simulink model "Series_Parallel_HEV_PowerFlow_Simulink"  (R2024b)
settings: Solver=VariableStepAuto  StartTime=0.0  StopTime=15  RelTol=1e-3
libraries: simulink x3
settings Model: Creator=JAMES  LastModifiedBy=JAMES

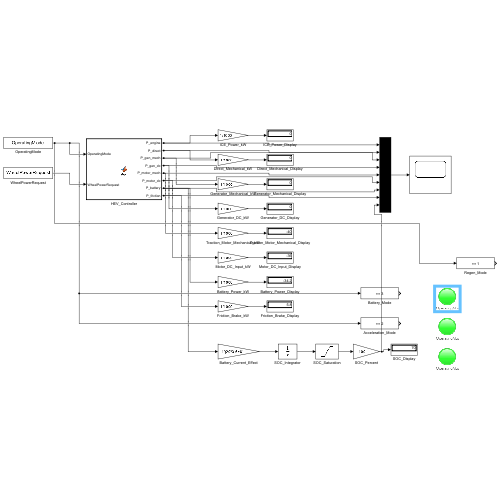
[thumbnail: Simulink's stored preview of the top-level diagram]
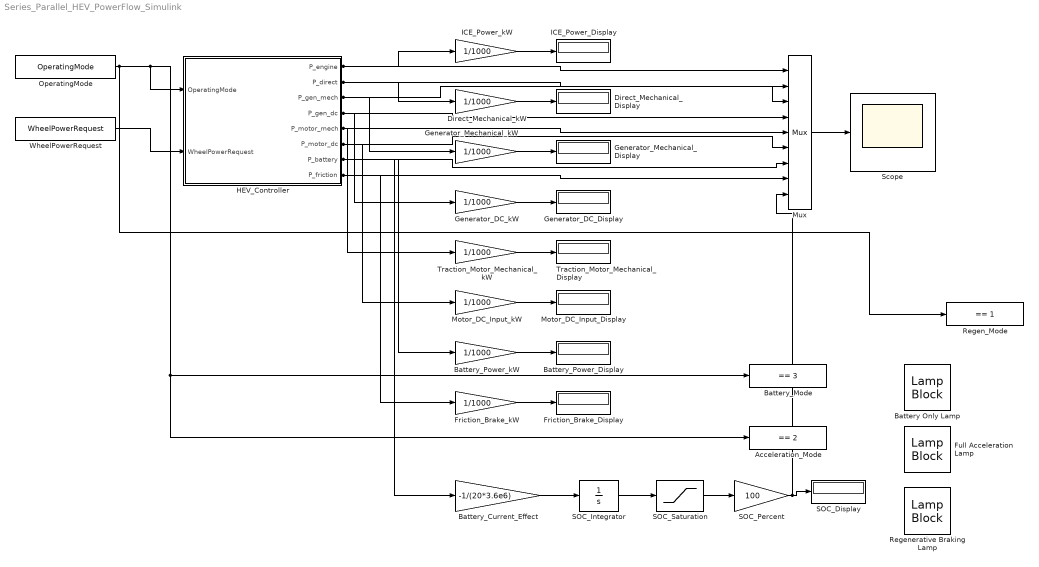
== system Series_Parallel_HEV_PowerFlow_Simulink ==
  Acceleration_Mode : simulink/Logic and Bit Operations/Compare To Constant  relop===  const=2  OutDataTypeStr=boolean
  Battery Only Lamp : LampBlock  LabelPosition=Bottom
  Battery_Current_Effect : Gain  Gain=-1/(20*3.6e6)
  Battery_Mode : simulink/Logic and Bit Operations/Compare To Constant  relop===  const=3  OutDataTypeStr=boolean
  Battery_Power_Display : Display
  Battery_Power_kW : Gain  Gain=1/1000
  Direct_Mechanical_Display : Display
  Direct_Mechanical_kW : Gain  Gain=1/1000
  Friction_Brake_Display : Display
  Friction_Brake_kW : Gain  Gain=1/1000
  Full Acceleration Lamp : LampBlock  LabelPosition=Bottom
  Generator_DC_Display : Display
  Generator_DC_kW : Gain  Gain=1/1000
  Generator_Mechanical_Display : Display
  Generator_Mechanical_kW : Gain  Gain=1/1000
  HEV_Controller : MATLAB Function  TreatAsAtomicUnit=on
  ICE_Power_Display : Display
  ICE_Power_kW : Gain  Gain=1/1000
  Motor_DC_Input_Display : Display
  Motor_DC_Input_kW : Gain  Gain=1/1000
  Mux : Mux  Inputs=9
  OperatingMode : FromWorkspace  VariableName=OperatingMode
  Regen_Mode : simulink/Logic and Bit Operations/Compare To Constant  relop===  const=1  OutDataTypeStr=boolean
  Regenerative Braking Lamp : LampBlock  LabelPosition=Bottom
  SOC_Display : Display
  SOC_Integrator : Integrator  InitialCondition=0.70
  SOC_Percent : Gain  Gain=100
  SOC_Saturation : Saturate  UpperLimit=1  LowerLimit=0
  Scope : Scope
  Traction_Motor_Mechanical_Display : Display
  Traction_Motor_Mechanical_kW : Gain  Gain=1/1000
  WheelPowerRequest : FromWorkspace  VariableName=WheelPowerRequest
  wires:
  ICE_Power_kW/1 -> ICE_Power_Display/1
  Direct_Mechanical_kW/1 -> Direct_Mechanical_Display/1
  Generator_Mechanical_kW/1 -> Generator_Mechanical_Display/1
  Generator_DC_kW/1 -> Generator_DC_Display/1
  Traction_Motor_Mechanical_kW/1 -> Traction_Motor_Mechanical_Display/1
  Motor_DC_Input_kW/1 -> Motor_DC_Input_Display/1
  Battery_Power_kW/1 -> Battery_Power_Display/1
  Friction_Brake_kW/1 -> Friction_Brake_Display/1
  OperatingMode/1 -> Battery_Mode/1, Acceleration_Mode/1, HEV_Controller/1(OperatingMode), Regen_Mode/1
  WheelPowerRequest/1 -> HEV_Controller/2(WheelPowerRequest)
  HEV_Controller/1(P_engine) -> ICE_Power_kW/1, Mux/1
  HEV_Controller/2(P_direct) -> Direct_Mechanical_kW/1, Mux/2
  HEV_Controller/3(P_gen_mech) -> Generator_Mechanical_kW/1, Mux/3
  HEV_Controller/4(P_gen_dc) -> Generator_DC_kW/1, Mux/4
  HEV_Controller/5(P_motor_mech) -> Traction_Motor_Mechanical_kW/1, Mux/5
  HEV_Controller/6(P_motor_dc) -> Motor_DC_Input_kW/1, Mux/6
  HEV_Controller/7(P_battery) -> Battery_Power_kW/1, Battery_Current_Effect/1, Mux/7
  HEV_Controller/8(P_friction) -> Friction_Brake_kW/1, Mux/8
  Battery_Current_Effect/1 -> SOC_Integrator/1
  SOC_Integrator/1 -> SOC_Saturation/1
  SOC_Saturation/1 -> SOC_Percent/1
  SOC_Percent/1 -> SOC_Display/1, Mux/9
  Mux/1 -> Scope/1

== matlab function Series_Parallel_HEV_PowerFlow_Simulink/HEV_Controller ==
  data: OperatingMode input; P_engine output; WheelPowerRequest input; P_direct output; P_gen_mech output; P_gen_dc output; P_motor_mech output; P_motor_dc output; P_battery output; P_friction output
function [P_engine,P_direct,P_gen_mech,P_gen_dc,P_motor_mech,P_motor_dc,P_battery,P_friction] = fcn(OperatingMode,WheelPowerRequest)

eta_engine = 0.90;
eta_generator = 0.90;
eta_motor = 0.90;
eta_battery = 0.95;

P_engine = 0;
P_direct = 0;
P_gen_mech = 0;
P_gen_dc = 0;
P_motor_mech = 0;
P_motor_dc = 0;
P_battery = 0;
P_friction = 0;

if OperatingMode == 3

    % Battery Only
    P_motor_mech = WheelPowerRequest;
    P_motor_dc = P_motor_mech / eta_motor;
    P_battery = P_motor_dc / eta_battery;

elseif OperatingMode == 2

    % Full Acceleration
    P_engine = WheelPowerRequest / eta_engine;
    P_direct = 0.5 * P_engine;

    P_gen_mech = P_engine - P_direct;
    P_gen_dc = P_gen_mech * eta_generator;

    P_motor_dc = P_gen_dc;
    P_motor_mech = P_motor_dc * eta_motor;

    P_battery = WheelPowerRequest - P_direct - P_motor_mech;

elseif OperatingMode == 1

    % Regenerative Braking
    braking_power = abs(WheelPowerRequest);

    P_motor_mech = -braking_power;
    P_motor_dc = P_motor_mech * eta_motor;

    P_battery = P_motor_dc * eta_battery;

    P_friction = braking_power - abs(P_battery);

end
